simulink model "drone_simulator"  (R2017a)
settings: Solver=FixedStepAuto  StartTime=0.0  StopTime=200  FixedStep=simulator.dt  RelTol=1e-3
undefined symbols (not defined in the file or in its folder): gnc_sub, simulator
settings Model: Creator=simone  LastModifiedBy=gcstation

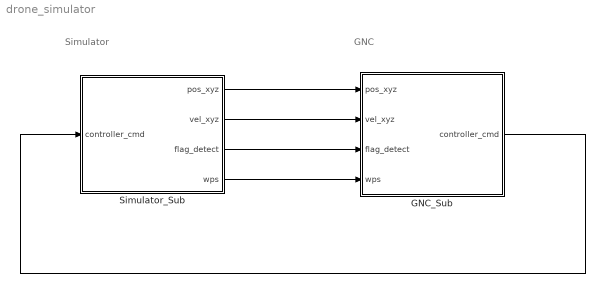
== system drone_simulator ==
  note: GNC
  note: Simulator
  GNC_Sub : Subsystem
  Simulator_Sub : Subsystem
  wires:
  Simulator_Sub/1(pos_xyz) -> GNC_Sub/1(pos_xyz)
  Simulator_Sub/2(vel_xyz) -> GNC_Sub/2(vel_xyz)
  GNC_Sub/1(controller_cmd) -> Simulator_Sub/1(controller_cmd)
  Simulator_Sub/3(flag_detect) -> GNC_Sub/3(flag_detect)
  Simulator_Sub/4(wps) -> GNC_Sub/4(wps)

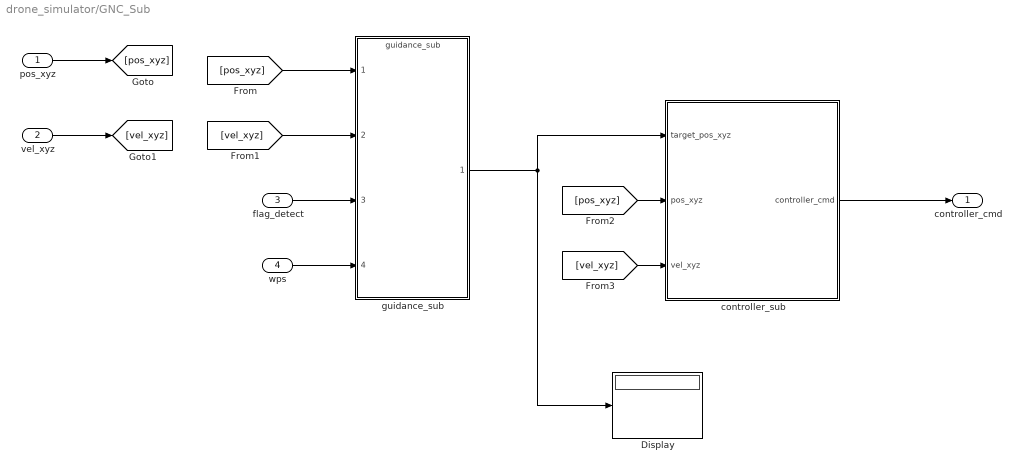
== system drone_simulator/GNC_Sub ==
  pos_xyz : Inport  PortDimensions=[3,1]
  vel_xyz : Inport  Port=2  PortDimensions=[3,1]
  flag_detect : Inport  Port=3  PortDimensions=[1,1]
  wps : Inport  Port=4
  Display : Display
  controller_sub : Subsystem
  guidance_sub : ModelReference  ModelNameDialog=guidance_sub  SimulationMode=Normal  ModelReferenceVersion=1.50
  controller_cmd : Outport
  wires:
  controller_sub/1(controller_cmd) -> controller_cmd/1
  flag_detect/1 -> guidance_sub/3
  guidance_sub/1 -> controller_sub/1(target_pos_xyz), Display/1
  [vel_xyz] -> controller_sub/3(vel_xyz)
  [pos_xyz] -> controller_sub/2(pos_xyz)
  pos_xyz/1 -> [pos_xyz]
  vel_xyz/1 -> [vel_xyz]
  [pos_xyz] -> guidance_sub/1
  [vel_xyz] -> guidance_sub/2
  wps/1 -> guidance_sub/4

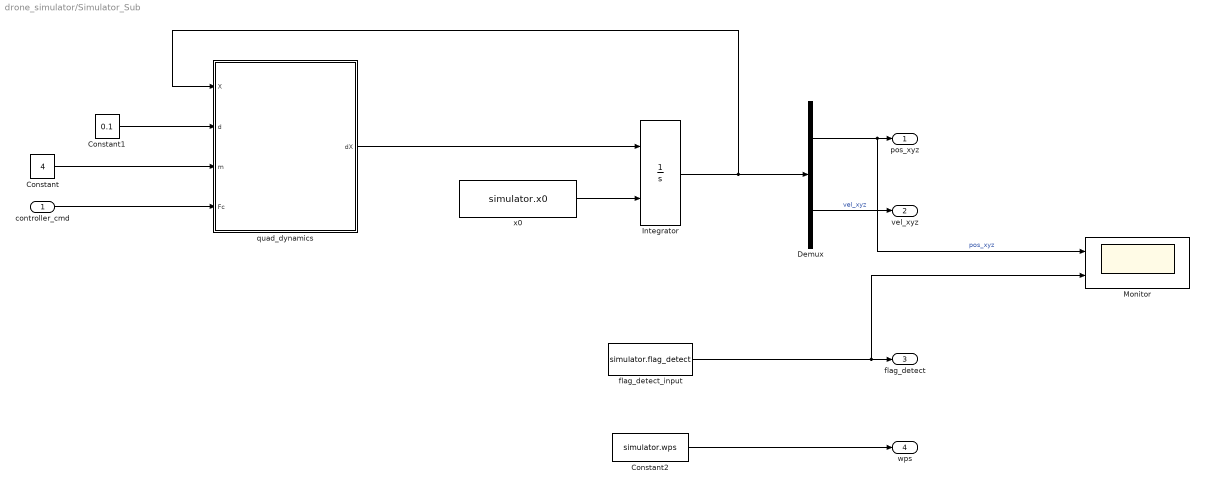
== system drone_simulator/Simulator_Sub ==
  controller_cmd : Inport
  Constant : Constant  Value=4
  Constant1 : Constant  Value=0.1
  Constant2 : Constant  Value=simulator.wps
  Demux : Demux  Outputs=2
  Integrator : Integrator  InitialConditionSource=external
  Monitor : Scope  NumInputPorts=2
  flag_detect_input : FromWorkspace  VariableName=simulator.flag_detect  SampleTime=0  Interpolate=off  OutputAfterFinalValue=Holding final value
  quad_dynamics : MATLAB Function  TreatAsAtomicUnit=on
  x0 : Constant  Value=simulator.x0
  pos_xyz : Outport
  vel_xyz : Outport  Port=2
  flag_detect : Outport  Port=3
  wps : Outport  Port=4
  wires:
  quad_dynamics/1(dX) -> Integrator/1
  Integrator/1 -> quad_dynamics/1(X), Demux/1
  Demux/1 -> Monitor/1, pos_xyz/1  "pos_xyz"
  Demux/2 -> vel_xyz/1  "vel_xyz"
  controller_cmd/1 -> quad_dynamics/4(Fc)
  Constant/1 -> quad_dynamics/3(m)
  Constant1/1 -> quad_dynamics/2(d)
  x0/1 -> Integrator/2
  flag_detect_input/1 -> Monitor/2, flag_detect/1
  Constant2/1 -> wps/1

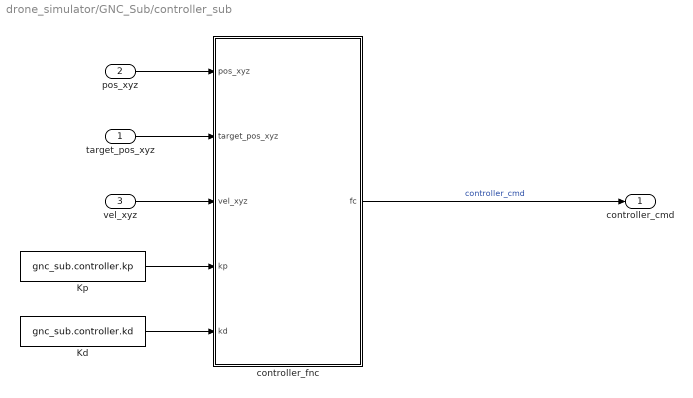
== system drone_simulator/GNC_Sub/controller_sub ==
  target_pos_xyz : Inport
  pos_xyz : Inport  Port=2
  vel_xyz : Inport  Port=3
  Kd : Constant  Value=gnc_sub.controller.kd
  Kp : Constant  Value=gnc_sub.controller.kp
  controller_fnc : MATLAB Function  TreatAsAtomicUnit=on
  controller_cmd : Outport
  wires:
  controller_fnc/1(fc) -> controller_cmd/1  "controller_cmd"
  Kp/1 -> controller_fnc/4(kp)
  Kd/1 -> controller_fnc/5(kd)
  target_pos_xyz/1 -> controller_fnc/2(target_pos_xyz)
  pos_xyz/1 -> controller_fnc/1(pos_xyz)
  vel_xyz/1 -> controller_fnc/3(vel_xyz)

== matlab function drone_simulator/Simulator_Sub/quad_dynamics ==
  data: X input; dX output; d input; m input; Fc input
function dX = quad_dynamics_wrp(X,d,m,Fc)
% X = [x,y,z,vx,vy,vz]'

dx = [X(4)
      X(5)
      X(6)];
ddx = -d*dx/m + Fc/m;

dX = [dx
      ddx];

end

== matlab function drone_simulator/GNC_Sub/controller_sub/controller_fnc ==
  data: pos_xyz input; fc output; target_pos_xyz input; vel_xyz input; kp input; kd input
function fc = fcn(pos_xyz, target_pos_xyz,vel_xyz,kp,kd)

fc = -kp*(pos_xyz-target_pos_xyz) - kd*(vel_xyz);
end
